simulink model "model_6ws6wd_SMC_ESO_final"  (R2023a)
settings: Solver=VariableStepAuto  StartTime=0.0  StopTime=20  RelTol=1e-3
libraries: slpidlib x2
settings Model: Creator=NGOC MAI  LastModifiedBy=NGOC MAI

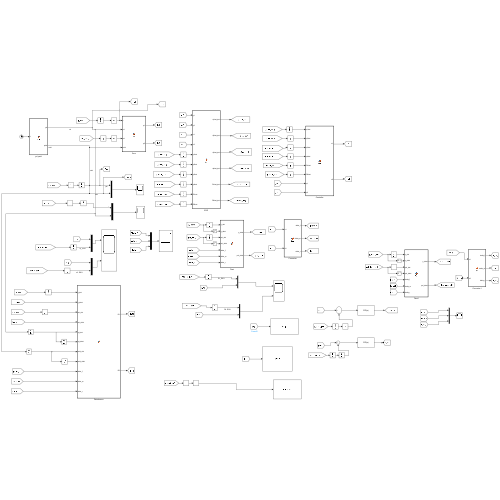
[thumbnail: Simulink's stored preview of the top-level diagram]
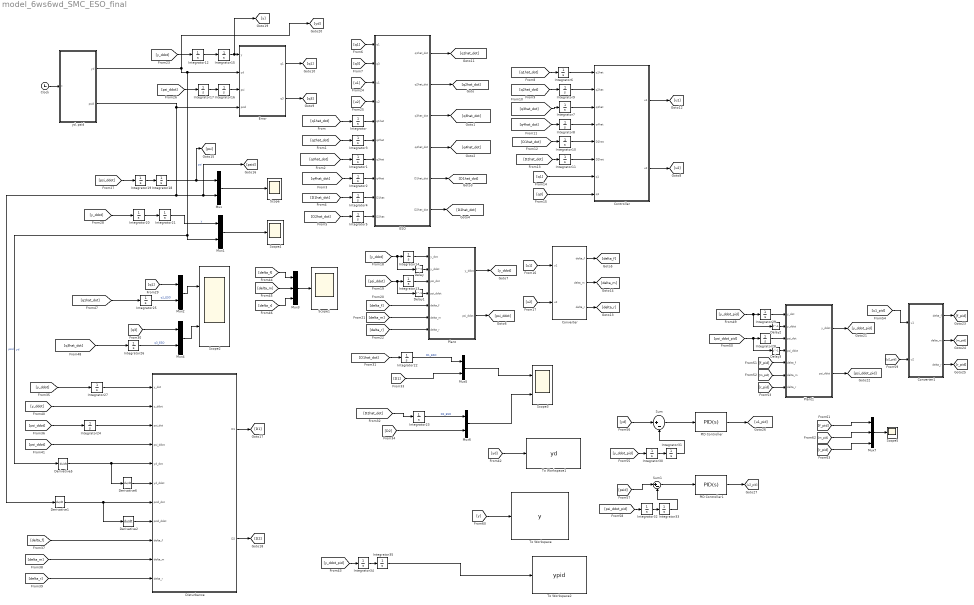
== system model_6ws6wd_SMC_ESO_final ==
  Clock : Clock
      settings: Decimation=20
  Controller : MATLAB Function  TreatAsAtomicUnit=on
  Converter : MATLAB Function  TreatAsAtomicUnit=on
  Converter1 : MATLAB Function  TreatAsAtomicUnit=on
  Delay{,1..3} (4 alike) : Delay  DelayLength=1
  Derivative{1..2,5..6} (4 alike) : Derivative
  Disturbance : MATLAB Function  TreatAsAtomicUnit=on
  ESO : MATLAB Function  TreatAsAtomicUnit=on
  Error : MATLAB Function  TreatAsAtomicUnit=on
  Integrator{,1..35} (36 alike) : Integrator
  Mux{,1..2,4..6} (6 alike) : Mux  Inputs=2
  Mux3 : Mux  Inputs=3
  Mux7 : Mux  Inputs=3
  PID Controller : slpidlib/PID Controller  Controller=PID  Form=Parallel  TimeDomain=Continuous-time  UseExternalTs=off  SampleTime=-1  IntegratorMethod=Forward Euler  FilterMethod=Forward Euler  ControllerParametersSource=internal  P=15  I=3  UseKiTs=off  D=5  N=100  UseFilter=on  TunerSelectOption=Transfer Function Based (PID Tuner App)  InitialConditionSource=internal  InitialConditionForIntegrator=0  InitialConditionForFilter=0  DifferentiatorICPrevScaledInput=0  ExternalReset=none  TrackingMode=off  Kt=1  LimitOutput=off  SatLimitsSource=internal  UpperSaturationLimit=inf  LowerSaturationLimit=-inf  LinearizeAsGain=on  AntiWindupMode=none  Kb=1  LimitIntegrator=off  UpperIntegratorSaturationLimit=inf  LowerIntegratorSaturationLimit=-inf  POutMin=[]  POutMax=[]  IOutMin=[]  IOutMax=[]  DOutMin=[]  DOutMax=[]  NOutMin=[]  NOutMax=[]  SumOutMin=[]  SumOutMax=[]  SaturationOutMin=[]  SaturationOutMax=[]  PParamMin=[]  PParamMax=[]  IParamMin=[]  IParamMax=[]  DParamMin=[]  DParamMax=[]  NParamMin=[]  NParamMax=[]  KbParamMin=[]  KbParamMax=[]  KtParamMin=[]  KtParamMax=[]  KbOutMin=[]  KbOutMax=[]  KtOutMin=[]  KtOutMax=[]  IntegratorOutMin=[]  IntegratorOutMax=[]  FilterOutMin=[]  FilterOutMax=[]  SumI1OutMin=[]  SumI1OutMax=[]  SumI2OutMin=[]  SumI2OutMax=[]  SumI3OutMin=[]  SumI3OutMax=[]  SumI4OutMin=[]  SumI4OutMax=[]  SumDOutMin=[]  SumDOutMax=[]  DifferentiatorOutMin=[]  DifferentiatorOutMax=[]  FilterDiffOutCoefMin=[]  FilterDiffOutCoefMax=[]  ReciprocalOutMin=[]  ReciprocalOutMax=[]  SumDenOutMin=[]  SumDenOutMax=[]  SumNumOutMin=[]  SumNumOutMax=[]  DivideOutMin=[]  DivideOutMax=[]  UdiffTsProdOutMin=[]  UdiffTsProdOutMax=[]  NTsProdOutMin=[]  NTsProdOutMax=[]  UintegralTsProdOutMin=[]  UintegralTsProdOutMax=[]  UngainTsProdOutMin=[]  UngainTsProdOutMax=[]  ClampingZeroOutDataTypeStr=Inherit: Inherit via back propagation  ClampingZeroOutMin=[]  ClampingZeroOutMax=[]  FilterDenConstantOutDataTypeStr=Inherit: Inherit via back propagation  FilterDenConstantOutMin=[]  FilterDenConstantOutMax=[]  PCopyOutDataTypeStr=Inherit: Inherit via back propagation  PCopyOutMin=[]  PCopyOutMax=[]  NCopyOutDataTypeStr=Inherit: Inherit via back propagation  NCopyOutMin=[]  NCopyOutMax=[]  IntegratorContinuousStateAttributes=''  IntegratorStateMustResolveToSignalObject=off  IntegratorRTWStateStorageClass=Auto  FilterContinuousStateAttributes=''  FilterStateMustResolveToSignalObject=off  FilterRTWStateStorageClass=Auto  ParallelPVariant=InternalParameters  IdealPVariant=Disabled  IVariant=InternalParameters  DVariant=InternalParameters  IntegratorVariant=Continuous  SatVariant=Disabled  AWVariant=Passthrough  PCopyVariant=Disabled  TRVariant=Disabled  FdbkBlocksVariant=Forward  IdealPFdbkVariant=Disabled  SatFdbkVariant=Disabled  DerivativeFilterVariant=ContFilter  NVariant=InternalParameters  NCopyVariant=Disabled  FilterICVariant=InternalICsFilter  IntegratorICVariant=InternalICs  ExternalResetVariant=Disabled  TRSumVariant=Passthrough  SumFdbkVariant=Disabled  SumVariant=Sum_PID  TsampFilterVariant=InternalTs  TsampNgainVariant=Passthrough  TsampIntegralVariant=Disabled_SignalSpec  ExternalSaturationOutDataTypeStr=Inherit: Same as second input
  PID Controller1 : slpidlib/PID Controller  Controller=PID  Form=Parallel  TimeDomain=Continuous-time  UseExternalTs=off  SampleTime=-1  IntegratorMethod=Forward Euler  FilterMethod=Forward Euler  ControllerParametersSource=internal  P=1700  I=20  UseKiTs=off  D=20  N=100  UseFilter=on  TunerSelectOption=Transfer Function Based (PID Tuner App)  InitialConditionSource=internal  InitialConditionForIntegrator=0  InitialConditionForFilter=0  DifferentiatorICPrevScaledInput=0  ExternalReset=none  TrackingMode=off  Kt=1  LimitOutput=off  SatLimitsSource=internal  UpperSaturationLimit=inf  LowerSaturationLimit=-inf  LinearizeAsGain=on  AntiWindupMode=none  Kb=1  LimitIntegrator=off  UpperIntegratorSaturationLimit=inf  LowerIntegratorSaturationLimit=-inf  POutMin=[]  POutMax=[]  IOutMin=[]  IOutMax=[]  DOutMin=[]  DOutMax=[]  NOutMin=[]  NOutMax=[]  SumOutMin=[]  SumOutMax=[]  SaturationOutMin=[]  SaturationOutMax=[]  PParamMin=[]  PParamMax=[]  IParamMin=[]  IParamMax=[]  DParamMin=[]  DParamMax=[]  NParamMin=[]  NParamMax=[]  KbParamMin=[]  KbParamMax=[]  KtParamMin=[]  KtParamMax=[]  KbOutMin=[]  KbOutMax=[]  KtOutMin=[]  KtOutMax=[]  IntegratorOutMin=[]  IntegratorOutMax=[]  FilterOutMin=[]  FilterOutMax=[]  SumI1OutMin=[]  SumI1OutMax=[]  SumI2OutMin=[]  SumI2OutMax=[]  SumI3OutMin=[]  SumI3OutMax=[]  SumI4OutMin=[]  SumI4OutMax=[]  SumDOutMin=[]  SumDOutMax=[]  DifferentiatorOutMin=[]  DifferentiatorOutMax=[]  FilterDiffOutCoefMin=[]  FilterDiffOutCoefMax=[]  ReciprocalOutMin=[]  ReciprocalOutMax=[]  SumDenOutMin=[]  SumDenOutMax=[]  SumNumOutMin=[]  SumNumOutMax=[]  DivideOutMin=[]  DivideOutMax=[]  UdiffTsProdOutMin=[]  UdiffTsProdOutMax=[]  NTsProdOutMin=[]  NTsProdOutMax=[]  UintegralTsProdOutMin=[]  UintegralTsProdOutMax=[]  UngainTsProdOutMin=[]  UngainTsProdOutMax=[]  ClampingZeroOutDataTypeStr=Inherit: Inherit via back propagation  ClampingZeroOutMin=[]  ClampingZeroOutMax=[]  FilterDenConstantOutDataTypeStr=Inherit: Inherit via back propagation  FilterDenConstantOutMin=[]  FilterDenConstantOutMax=[]  PCopyOutDataTypeStr=Inherit: Inherit via back propagation  PCopyOutMin=[]  PCopyOutMax=[]  NCopyOutDataTypeStr=Inherit: Inherit via back propagation  NCopyOutMin=[]  NCopyOutMax=[]  IntegratorContinuousStateAttributes=''  IntegratorStateMustResolveToSignalObject=off  IntegratorRTWStateStorageClass=Auto  FilterContinuousStateAttributes=''  FilterStateMustResolveToSignalObject=off  FilterRTWStateStorageClass=Auto  ParallelPVariant=InternalParameters  IdealPVariant=Disabled  IVariant=InternalParameters  DVariant=InternalParameters  IntegratorVariant=Continuous  SatVariant=Disabled  AWVariant=Passthrough  PCopyVariant=Disabled  TRVariant=Disabled  FdbkBlocksVariant=Forward  IdealPFdbkVariant=Disabled  SatFdbkVariant=Disabled  DerivativeFilterVariant=ContFilter  NVariant=InternalParameters  NCopyVariant=Disabled  FilterICVariant=InternalICsFilter  IntegratorICVariant=InternalICs  ExternalResetVariant=Disabled  TRSumVariant=Passthrough  SumFdbkVariant=Disabled  SumVariant=Sum_PID  TsampFilterVariant=InternalTs  TsampNgainVariant=Passthrough  TsampIntegralVariant=Disabled_SignalSpec  ExternalSaturationOutDataTypeStr=Inherit: Same as second input
  Plant : MATLAB Function  TreatAsAtomicUnit=on
  Plant1 : MATLAB Function  TreatAsAtomicUnit=on
  Scope{,1,4..5} (4 alike) : Scope
  Scope2 : Scope  NumInputPorts=2
  Scope3 : Scope  NumInputPorts=2
  Sum : Sum  Inputs=|+-
  Sum1 : Sum  Inputs=|+-
  To Workspace : ToWorkspace  VariableName=y  SaveFormat=Timeseries  SampleTime=-1
  To Workspace1 : ToWorkspace  VariableName=yd  SaveFormat=Timeseries  SampleTime=-1
  To Workspace2 : ToWorkspace  VariableName=ypid  SaveFormat=Timeseries  SampleTime=-1
  "yd, psid" : MATLAB Function  TreatAsAtomicUnit=on
  wires:
  Clock/1 -> "yd, psid"/1(t)
  ESO/5(D1hat_dot) -> [D1hat_dot]
  ESO/6(D2hat_dot) -> [D2hat_dot]
  ESO/4(q4hat_dot) -> [q4hat_dot]
  ESO/3(q3hat_dot) -> [q3hat_dot]
  ESO/2(q2hat_dot) -> [q2hat_dot]
  ESO/1(q1hat_dot) -> [q1hat_dot]
  Integrator/1 -> ESO/5(q1hat)
  Integrator3/1 -> ESO/6(q2hat)
  Integrator1/1 -> ESO/7(q3hat)
  Integrator2/1 -> ESO/8(q4hat)
  [q1hat_dot] -> Integrator/1
  [q3hat_dot] -> Integrator1/1
  [q2hat_dot] -> Integrator3/1
  [q4hat_dot] -> Integrator2/1
  Integrator5/1 -> ESO/10(D2hat)
  Integrator4/1 -> ESO/9(D1hat)
  [D1hat_dot] -> Integrator4/1
  [D2hat_dot] -> Integrator5/1
  [q1] -> ESO/1(q1)
  [q3] -> ESO/2(q3)
  "yd, psid"/1(yd) -> Error/2(yd), Derivative5/1, Mux1/2, [yd]  "yd"
  Integrator11/1 -> Controller/6(D2hat)
  Integrator6/1 -> Controller/1(q1hat)
  [D1hat_dot] -> Integrator10/1
  [q4hat_dot] -> Integrator8/1
  Integrator10/1 -> Controller/5(D1hat)
  Integrator8/1 -> Controller/4(q4hat)
  [q1hat_dot] -> Integrator6/1
  [D2hat_dot] -> Integrator11/1
  [q2hat_dot] -> Integrator9/1
  Integrator9/1 -> Controller/2(q2hat)
  [q1] -> Controller/7(q1)
  [q3] -> Controller/8(q3)
  Controller/1(u1) -> [u1]
  Controller/2(u2) -> [u2]
  [u1] -> Converter/1(u1)
  [u2] -> Converter/2(u2)
  Integrator14/1 -> Plant/1(y_dot)
  [y_ddot] -> Delay/1, Integrator14/1
  [psi_ddot] -> Delay1/1, Integrator13/1
  Integrator13/1 -> Plant/3(psi_dot)
  Plant/1(y_ddot) -> [y_ddot]
  Plant/2(psi_ddot) -> [psi_ddot]
  Converter/1(delta_f) -> [delta_f]
  Converter/2(delta_m) -> [delta_m]
  Converter/3(delta_r) -> [delta_r]
  [delta_f] -> Plant/5(delta_f)
  [delta_m] -> Plant/6(delta_m)
  [delta_r] -> Plant/7(delta_r)
  [y_ddot] -> Integrator12/1
  [u1] -> ESO/3(u1)
  [u2] -> ESO/4(u2)
  [psi_ddot] -> Integrator17/1
  Integrator17/1 -> Integrator16/1
  Integrator16/1 -> Error/3(psi)
  [psi_ddot] -> Integrator19/1
  Integrator19/1 -> Integrator18/1
  [y_ddot] -> Integrator20/1
  Integrator18/1 -> [psi], Mux/1  "psi"
  Integrator21/1 -> Mux1/1  "y"
  Mux/1 -> Scope/1
  [q1] -> Mux2/1
  "yd, psid"/2(psid) -> [psid], Mux/2, Derivative1/1, Error/4(psid)  "psid"
  [delta_f] -> Mux3/1
  [delta_m] -> Mux3/2
  [delta_r] -> Mux3/3
  Mux3/1 -> Scope1/1
  Integrator25/1 -> Mux2/2  "q1_ESO"
  [q1hat_dot] -> Integrator25/1
  Mux2/1 -> Scope2/1
  Mux4/1 -> Scope2/2
  Integrator20/1 -> Integrator21/1
  Error/2(q3) -> [q3]
  [D1hat_dot] -> Integrator22/1
  [D2hat_dot] -> Integrator23/1
  Disturbance/1(D1) -> [D1]
  [delta_f] -> Disturbance/9(delta_f)
  [delta_r] -> Disturbance/11(delta_r)
  Integrator27/1 -> Disturbance/1(y_dot)
  [delta_m] -> Disturbance/10(delta_m)
  [psi_ddot] -> Integrator24/1
  Disturbance/2(D2) -> [D2]
  [y_ddot] -> Integrator27/1
  Integrator24/1 -> Disturbance/3(psi_dot)
  Derivative2/1 -> Disturbance/8(psid_ddot)
  Derivative1/1 -> Derivative2/1, Disturbance/7(psid_dot)
  [y_ddot] -> Disturbance/2(y_ddot)
  [psi_ddot] -> Disturbance/4(psi_ddot)
  Integrator22/1 -> Mux5/1  "D1_ESO"
  Mux5/1 -> Scope3/1
  Integrator23/1 -> Mux6/1  "D2_ESO"
  Mux6/1 -> Scope3/2
  Mux1/1 -> Scope4/1
  Derivative6/1 -> Disturbance/6(yd_ddot)
  Derivative5/1 -> Disturbance/5(yd_dot), Derivative6/1
  Integrator7/1 -> Controller/3(q3hat)
  [q3hat_dot] -> Integrator7/1
  [D1] -> Mux5/2
  [D2] -> Mux6/2
  Delay1/1 -> Plant/4("psi_ddot ")
  Delay/1 -> Plant/2("y_ddot ")
  Error/1(q1) -> [q1]
  Integrator12/1 -> Integrator15/1
  Integrator15/1 -> [y], Error/1(y)
  [q3] -> Mux4/1
  [q3hat_dot] -> Integrator26/1
  Integrator26/1 -> Mux4/2  "q3_ESO"
  Integrator29/1 -> Plant1/1(y_dot)
  Delay3/1 -> Plant1/4("psi_ddot ")
  [y_ddot_pid] -> Delay2/1, Integrator29/1
  Plant1/1(y_ddot) -> [y_ddot_pid]
  Delay2/1 -> Plant1/2("y_ddot ")
  Converter1/1(delta_f) -> [f_pid]
  Plant1/2(psi_ddot) -> [psi_ddot_pid]
  Converter1/3(delta_r) -> [r_pid]
  Integrator28/1 -> Plant1/3(psi_dot)
  Converter1/2(delta_m) -> [m_pid]
  [psi_ddot_pid] -> Delay3/1, Integrator28/1
  [f_pid] -> Plant1/5(delta_f)
  [m_pid] -> Plant1/6(delta_m)
  [r_pid] -> Plant1/7(delta_r)
  [yd] -> Sum/1
  Sum/1 -> PID Controller/1
  PID Controller/1 -> [u1_pid]
  [u1_pid] -> Converter1/1(u1)
  [y_ddot_pid] -> Integrator30/1
  Integrator30/1 -> Integrator31/1
  Integrator31/1 -> Sum/2
  [psid] -> Sum1/1
  Sum1/1 -> PID Controller1/1
  [psi_ddot_pid] -> Integrator32/1
  Integrator32/1 -> Integrator33/1
  Integrator33/1 -> Sum1/2
  PID Controller1/1 -> [u2_pid]
  [u2_pid] -> Converter1/2(u2)
  [m_pid] -> Mux7/2
  [r_pid] -> Mux7/3
  [f_pid] -> Mux7/1
  Mux7/1 -> Scope5/1
  [yd] -> To Workspace1/1
  [y_ddot_pid] -> Integrator34/1
  Integrator34/1 -> Integrator35/1
  Integrator35/1 -> To Workspace2/1
  [y] -> To Workspace/1

== matlab function model_6ws6wd_SMC_ESO_final/Disturbance ==
  data: y_dot input; y_ddot input; psi_dot input; psi_ddot input; yd_dot input; yd_ddot input; psid_dot input; psid_ddot input; delta_f input; delta_m input; delta_r input; D1 output; D2 output
function [D1, D2] = fcn(y_dot, y_ddot, psi_dot, psi_ddot, yd_dot, yd_ddot, psid_dot, psid_ddot, delta_f, delta_m, delta_r)
m = 8800; %kg
J = 1350; %kgm^2
cf = 55000; %N/rad
cm = 100000; %N/rad
cr = 120000; %N/rad
lf = 1.95; %m
lm = 0.1; %m
lr = 1.95; %m
vx = 20; %m/s

g = 9.8; %m/s^2
theta = 0.087; %rad

cf_t = 2000; %N/rad
cm_t = 3000; %N/rad
cr_t = 5000; %N/rad
m_t = 150; %kg
J_t = 60; %kgm^2
M = m_t + m;

a1 = -2*(cf + cm + cr)/(m*vx);
a2 = -2*(lf*cf - lr*cr + lm*cm)/(m*vx) - vx;
n1 = -2*(lf*cf - lr*cr + lm*cm)/(J*vx);
n2 = -2*((lf^2)*cf + (lr^2)*cr + (lm^2)*cm)/(J*vx);

%k1=2*(-cf-cr-cm)/(m*vx);
%k3=2*(cf+cr+cm)/m;
%k2=-2*(lf*cf-lr*cr+lm*cm)/(m*vx);
%k4=2*(-lf*cf+lr*cr-lm*cm)/(J*vx);
%k6=2*(lf*cf-lr*cr+lm*cm)/J;
%k5=-2*((lf^2)*cf+(lm^2)*cm+(lr^2)*cr)/(J*vx);

d1 = (-2*(cf_t + cm_t + cr_t)/(m*vx))*y_dot + (-2*(cf_t*lf + cm_t*lm - cr_t*lr)/(m*vx) - m_t*vx/m)*psi_dot + 2*(cf_t*delta_f + cm_t*delta_m + cr_t*delta_r)/m + M*g*sin(theta)/m - m_t*y_ddot/m;
d2 = (-2*(lf*cf_t + lm*cm_t - lr*cr_t)/(J*vx))*y_dot + (-2*(cf_t*lf^2 + cm_t*lm^2 + cr_t*lr^2)/(J*vx))*psi_dot + 2*(lf*cf_t*delta_f + lm*cm_t*delta_m - lr*cr_t*delta_r)/J - J_t*psi_ddot/J; 

D1 = a1*yd_dot + a2*psid_dot + d1 - yd_ddot; 
D2 = n1*yd_dot + n2*psid_dot + d2 - psid_ddot;

end

== matlab function model_6ws6wd_SMC_ESO_final/Converter1 ==
  data: u1 input; delta_f output; u2 input; delta_m output; delta_r output
function [delta_f,delta_m,delta_r] = fcn(u1,u2)
m=8800; %kg
J=1350; %kgm^2
cf=55000; %N/rad
cm=100000; %N/rad
cr=120000; %N/rad
lf=1.95; %m
lm=0.1; %m
lr=1.95; %m
%vx=20; %m/s
A=[cf cm cr;cf*lf cm*lm -cr*lr;1/2 -1 1/2];
B=[u1*m/2;u2*J/2;0];
C=A^(-1)*B;
delta_f=C(1,1);
delta_m=C(2,1);
delta_r=C(3,1);
end

== matlab function model_6ws6wd_SMC_ESO_final/Plant1 ==
  data: y_dot input; y_ddot input; y_ddot output; psi_dot input; psi_ddot input; delta_f input; delta_m input; psi_ddot output; delta_r input
function [y_ddot, psi_ddot] = fcn(y_dot, y_ddot, psi_dot, psi_ddot, delta_f, delta_m, delta_r)
m = 8800; %kg
J = 1350; %kgm^2
cf = 55000; %N/rad
cm = 100000; %N/rad
cr = 120000; %N/rad
lf = 1.95; %m
lm = 0.1; %m
lr = 1.95; %m
vx = 20; %m/s

g = 9.8; %m/s^2
theta = 0.087; %rad

cf_t = 2000; %N/rad
cm_t = 3000; %N/rad
cr_t = 5000; %N/rad
m_t = 150; %kg
J_t = 60; %kgm^2
M = m_t + m;

m1 = -2*(cf + cm + cr)/(m*vx);
m2 = -2*(lf*cf - lr*cr + lm*cm)/(m*vx) - vx;
n1 = -2*(lf*cf - lr*cr + lm*cm)/(J*vx);
n2 = -2*((lf^2)*cf + (lr^2)*cr + (lm^2)*cm)/(J*vx);

d1 = (-2*(cf_t + cm_t + cr_t)/(m*vx))*y_dot + (-2*(cf_t*lf + cm_t*lm - cr_t*lr)/(m*vx) - m_t*vx/m)*psi_dot + 2*(cf_t*delta_f + cm_t*delta_m + cr_t*delta_r)/m + M*g*sin(theta)/m - m_t*y_ddot/m;
d2 = (-2*(lf*cf_t + lm*cm_t - lr*cr_t)/(J*vx))*y_dot + (-2*(cf_t*lf^2 + cm_t*lm^2 + cr_t*lr^2)/(J*vx))*psi_dot + 2*(lf*cf_t*delta_f + lm*cm_t*delta_m - lr*cr_t*delta_r)/J - J_t*psi_ddot/J; 

u1 = 2*(cf*delta_f + cm*delta_m + cr*delta_r)/m;
u2 = 2*(lf*cf*delta_f + lm*cm*delta_m - lr*cr*delta_r)/J;
y_ddot = m1*y_dot + m2*psi_dot + u1 + d1;
psi_ddot = n1*y_dot + n2*psi_dot + u2 + d2 ;
end

== matlab function model_6ws6wd_SMC_ESO_final/Error ==
  data: y input; yd input; q1 output; psi input; psid input; q3 output
function [q1,q3]= fcn(y,yd,psi,psid)
q1=y-yd;
q3=psi-psid;
end

%function [q1dot,q3]= fcn(y_dot,psi,psid)
%q1dot = y_dot + 20*(psi - psid);
%q3 = psi - psid;
%end

== matlab function model_6ws6wd_SMC_ESO_final/Plant ==
  data: y_dot input; y_ddot input; y_ddot output; psi_dot input; psi_ddot input; delta_f input; delta_m input; psi_ddot output; delta_r input
function [y_ddot, psi_ddot] = fcn(y_dot, y_ddot, psi_dot, psi_ddot, delta_f, delta_m, delta_r)
m = 8800; %kg
J = 1350; %kgm^2
cf = 55000; %N/rad
cm = 100000; %N/rad
cr = 120000; %N/rad
lf = 1.95; %m
lm = 0.1; %m
lr = 1.95; %m
vx = 20; %m/s

g = 9.8; %m/s^2
theta = 0.087; %rad

cf_t = 2000; %N/rad
cm_t = 3000; %N/rad
cr_t = 5000; %N/rad
m_t = 150; %kg
J_t = 60; %kgm^2
M = m_t + m;

m1 = -2*(cf + cm + cr)/(m*vx);
m2 = -2*(lf*cf - lr*cr + lm*cm)/(m*vx) - vx;
n1 = -2*(lf*cf - lr*cr + lm*cm)/(J*vx);
n2 = -2*((lf^2)*cf + (lr^2)*cr + (lm^2)*cm)/(J*vx);

d1 = (-2*(cf_t + cm_t + cr_t)/(m*vx))*y_dot + (-2*(cf_t*lf + cm_t*lm - cr_t*lr)/(m*vx) - m_t*vx/m)*psi_dot + 2*(cf_t*delta_f + cm_t*delta_m + cr_t*delta_r)/m + M*g*sin(theta)/m - m_t*y_ddot/m;
d2 = (-2*(lf*cf_t + lm*cm_t - lr*cr_t)/(J*vx))*y_dot + (-2*(cf_t*lf^2 + cm_t*lm^2 + cr_t*lr^2)/(J*vx))*psi_dot + 2*(lf*cf_t*delta_f + lm*cm_t*delta_m - lr*cr_t*delta_r)/J - J_t*psi_ddot/J; 

u1 = 2*(cf*delta_f + cm*delta_m + cr*delta_r)/m;
u2 = 2*(lf*cf*delta_f + lm*cm*delta_m - lr*cr*delta_r)/J;
y_ddot = m1*y_dot + m2*psi_dot + u1 + d1;
psi_ddot = n1*y_dot + n2*psi_dot + u2 + d2 ;
end

== matlab function model_6ws6wd_SMC_ESO_final/ESO ==
  data: q1 input; q1hat_dot output; q3 input; u1 input; u2 input; q1hat input; q2hat input; q3hat input; q4hat input; D1hat input; D2hat input; q2hat_dot output; q3hat_dot output; q4hat_dot output; D1hat_dot output; D2hat_dot output
function [q1hat_dot,q2hat_dot,q3hat_dot,q4hat_dot,D1hat_dot,D2hat_dot]= fcn(q1,q3,u1,u2,q1hat,q2hat,q3hat,q4hat,D1hat,D2hat)
m = 8800; %kg
J = 1350; %kgm^2
cf = 55000; %N/rad
cm = 100000; %N/rad
cr = 120000; %N/rad
lf = 1.95; %m
lm = 0.1; %m
lr = 1.95; %m
vx = 20; %m/s

%k1 = 2*(-cf-cr-cm)/(m*vx);
%k3 = 2*(cf+cr+cm)/m;
%k2 = -2*(lf*cf-lr*cr+lm*cm)/(m*vx);
%k4 = 2*(-lf*cf+lr*cr-lm*cm)/(J*vx);
%k6 = 2*(lf*cf-lr*cr+lm*cm)/J;
%k5 = -2*((lf^2)*cf+(lm^2)*cm+(lr^2)*cr)/(J*vx);

m1 = -2*(cf + cm + cr)/(m*vx);
m2 = -2*(lf*cf - lr*cr + lm*cm)/(m*vx) - vx;
n1 = -2*(lf*cf - lr*cr + lm*cm)/(J*vx);
n2 = -2*((lf^2)*cf + (lr^2)*cr + (lm^2)*cm)/(J*vx);

a1 = 6;
a2 = 11;
a3 = 6;
epsi1 = 0.027;
epsi2 = 0.01;

q1hat_dot = q2hat + a1*(q1 - q1hat)/epsi1;
q2hat_dot = D1hat + m1*q2hat + m2*q4hat + u1 + a2*(q1 - q1hat)/(epsi1^2);
D1hat_dot = a3*(q1 - q1hat)/(epsi1^3);
q3hat_dot = q4hat + a1*(q3 - q3hat)/epsi2;
q4hat_dot = D2hat + n1*q2hat + n2*q4hat + u2 + a2*(q3 - q3hat)/(epsi2^2);
D2hat_dot = a3*(q3 - q3hat)/epsi2^3;
end

== matlab function model_6ws6wd_SMC_ESO_final/yd, psid ==
  data: t input; yd output; psid output
function [yd,psid]= fcn(t)
yd = 1.5*(tanh(t-6) - tanh(t-14));
psid = ((3*tanh(t - 14)^2)/2 - (3*tanh(t - 6)^2)/2)/20;
%psid = 1.5*(-(sech(t-14))^2 + (sech(t-6))^2)/20;
end

== matlab function model_6ws6wd_SMC_ESO_final/Controller ==
  data: u1 output; u2 output; q1hat input; q2hat input; q3hat input; q4hat input; D1hat input; D2hat input; q1 input; q3 input
function [u1, u2]= fcn(q1hat, q2hat, q3hat, q4hat, D1hat, D2hat, q1, q3)
a1 = 6;
a2 = 11;
%a3 = 6;
epsi1 = 0.027;
epsi2 = 0.01;
p1 = 12;
p2 = 25;
c1 = 3;
c2 = 0.5;
c3 = 2;
c4 = 4;

m = 8800; %kg
J = 1350; %kgm^2
cf = 55000; %N/rad
cm = 100000; %N/rad
cr = 120000; %N/rad
lf = 1.95; %m
lm = 0.1; %m
lr = 1.95; %m
vx = 20; %m/s

%k1 = 2*(-cf - cr - cm)/(m*vx);
%k3 = 2*(cf + cr + cm)/m;
%k2 = -2*(lf*cf - lr*cr + lm*cm)/(m*vx);
%k4 = 2*(-lf*cf + lr*cr - lm*cm)/(J*vx);
%k6 = 2*(lf*cf - lr*cr + lm*cm)/J;
%k5 = -2*((lf^2)*cf + (lm^2)*cm + (lr^2)*cr)/(J*vx);

m1 = -2*(cf + cm + cr)/(m*vx);
m2 = -2*(lf*cf - lr*cr + lm*cm)/(m*vx) - vx;
n1 = -2*(lf*cf - lr*cr + lm*cm)/(J*vx);
n2 = -2*((lf^2)*cf + (lr^2)*cr + (lm^2)*cm)/(J*vx);

s1 = p1*q1hat + q2hat;
s2 = p2*q3hat + q4hat;

u1 = -c1*s1 - c2*sat(s1) - p1*q2hat - p1*a1*(q1 - q1hat)/epsi1 - D1hat - m1*q2hat - m2*q4hat - a2*(q1 - q1hat)/epsi1^2;
u2 = -c3*s2 - c4*sat(s2) - p2*q4hat - p2*a1*(q3 - q3hat)/epsi2 - D2hat - n1*q2hat - n2*q4hat - a2*(q3 - q3hat)/epsi2^2;
end

== matlab function model_6ws6wd_SMC_ESO_final/Converter ==
  data: u1 input; delta_f output; u2 input; delta_m output; delta_r output
function [delta_f,delta_m,delta_r] = fcn(u1,u2)
m=8800; %kg
J=1350; %kgm^2
cf=55000; %N/rad
cm=100000; %N/rad
cr=120000; %N/rad
lf=1.95; %m
lm=0.1; %m
lr=1.95; %m
%vx=20; %m/s
A=[cf cm cr;cf*lf cm*lm -cr*lr;1/2 -1 1/2];
B=[u1*m/2;u2*J/2;0];
C=A^(-1)*B;
delta_f=C(1,1);
delta_m=C(2,1);
delta_r=C(3,1);
end
